simulink model "Week10_Simulation_Trajectory"  (R2017b)
settings: Solver=ode4  StartTime=0.0  StopTime=20  FixedStep=1e-3  RelTol=1e-3  EnableMultiTasking=on
undefined symbols (not defined in the file): DiscIntNeverNeededParam
libraries: simulink x2
settings Model: Creator=e27269  LastModifiedBy=e27269
settings DataIOCC: LimitDataPoints=on
settings OptimizationCC: LifeSpan=inf
settings DebuggingCC: AllowSymbolicDim=off  SFUnexpectedBacktrackingDiag=warning  SFNoUnconditionalDefaultTransitionDiag=warning  SFExecutionAtInitializationDiag=none
settings ModelReferenceCC: PropagateSignalLabelsOutOfModel=off
settings CodeAppCC: StateflowObjectComments=on
settings GRTTargetCC: TargetLangStandard=C89/C90 (ANSI)
settings ConfigComp: CovMetricSettings=dw  CovHtmlReporting=on  CovSaveCumulativeToWorkspaceVar=on  CovSaveSingleToWorkspaceVar=on  CovExternalEMLEnable=off

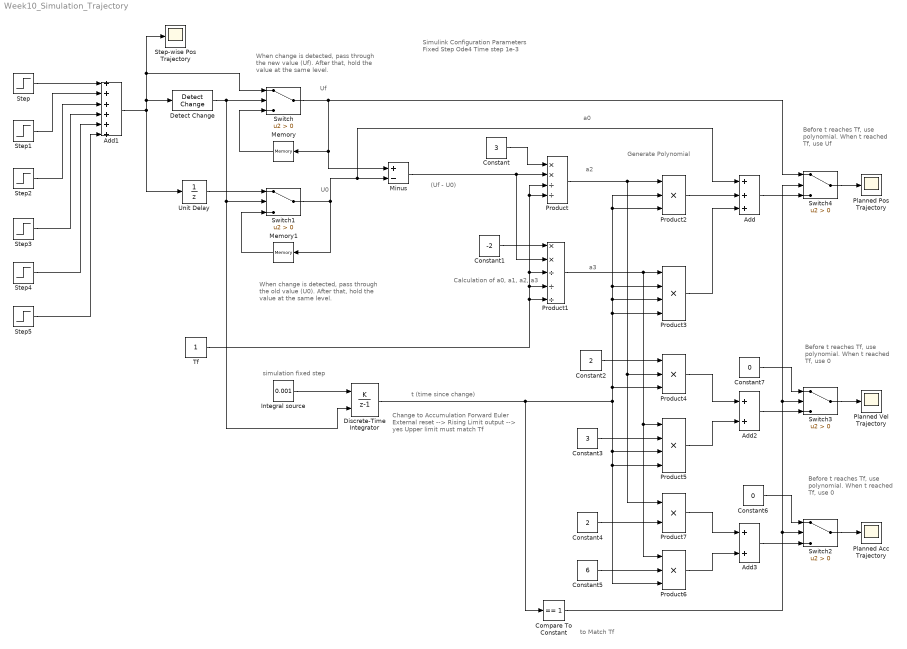
== system Week10_Simulation_Trajectory ==
  note: Generate Polynomial
  note: Calculation of
      | a0, a1, a2, a3
  note: Before t reaches Tf,
      | use polynomial.
      | When t reached Tf,
      | use Uf
  note: to Match Tf
  note: t (time since change)
  note: (Uf - U0)
  note: When change is detected, pass through
      | the old value (U0). After that, hold the
      | value at the same level.
  note: Simulink Configuration Parameters
      | Fixed Step
      | Ode4
      | Time step 1e-3
  note: simulation fixed step
  note: Change to Accumulation Forward Euler
      | External reset --> Rising
      | Limit output --> yes
      | Upper limit must match Tf
  note: a0
  note: a3
  note: a2
  note: Uf
  note: U0
  note: When change is detected, pass through
      | the new value (Uf). After that, hold the
      | value at the same level.
  note: Before t reaches Tf,
      | use polynomial.
      | When t reached Tf,
      | use 0
  note: Before t reaches Tf,
      | use polynomial.
      | When t reached Tf,
      | use 0
  Add : Sum  Inputs=3
  Add1 : Sum  Inputs=6
  Add2 : Sum  Inputs=2
  Add3 : Sum  Inputs=2
  Compare To Constant : simulink/Logic and Bit Operations/Compare To Constant  relop===  const=1  OutDataTypeStr=boolean
  Constant : Constant  Value=3
  Constant1 : Constant  Value=-2
  Constant2 : Constant  Value=2
  Constant3 : Constant  Value=3
  Constant4 : Constant  Value=2
  Constant5 : Constant  Value=6
  Constant6 : Constant  Value=0
  Constant7 : Constant  Value=0
  Detect Change : simulink/Logic and Bit Operations/Detect Change  vinit=0  InputProcessing=Inherited  OutDataTypeStr=boolean
  Discrete-Time Integrator : DiscreteIntegrator  IntegratorMethod=Accumulation: Forward Euler  gainval=1  ExternalReset=rising  InitialConditionSetting=State (most efficient)  SampleTime=-1  LimitOutput=on  UpperSaturationLimit=1  ICPrevOutput=DiscIntNeverNeededParam  ICPrevScaledInput=DiscIntNeverNeededParam
  Integral source : Constant  Value=0.001
  Memory : Memory  InheritSampleTime=on
  Memory1 : Memory  InheritSampleTime=on
  Minus : Sum  Inputs=+-
  Planned Acc Trajectory : Scope
  Planned Pos Trajectory : Scope
  Planned Vel Trajectory : Scope
  Product : Product  Inputs=**//
  Product1 : Product  Inputs=**///
  Product2 : Product  Inputs=3
  Product3 : Product  Inputs=4
  Product4 : Product  Inputs=3
  Product5 : Product  Inputs=4
  Product6 : Product  Inputs=3
  Product7 : Product
  Step : Step  SampleTime=0
  Step-wise Pos Trajectory : Scope
  Step1 : Step  Time=4  After=2  SampleTime=0
  Step2 : Step  Time=8  After=-1  SampleTime=0
  Step3 : Step  Time=11  After=1.5  SampleTime=0
  Step4 : Step  Time=14  After=-1  SampleTime=0
  Step5 : Step  Time=17  After=-2  SampleTime=0
  Switch{,1..4} (5 alike) : Switch  Criteria=u2 > Threshold
  Tf : Constant
  Unit Delay : UnitDelay  SampleTime=-1
  wires:
  Switch/1 -> Minus/1, Memory/1, Switch4/1
  Memory/1 -> Switch/3
  Unit Delay/1 -> Switch1/1
  Switch1/1 -> Memory1/1, Add/1, Minus/2
  Memory1/1 -> Switch1/3
  Minus/1 -> Product1/2, Product/2
  Constant/1 -> Product/1
  Tf/1 -> Product1/5, Product1/4, Product1/3, Product/4, Product/3
  Product/1 -> Product7/1, Product4/2, Product2/1
  Constant1/1 -> Product1/1
  Product1/1 -> Product6/1, Product5/1, Product3/1
  Integral source/1 -> Discrete-Time Integrator/1
  Discrete-Time Integrator/1 -> Compare To Constant/1, Product5/3, Product6/3, Product5/4, Product4/3, Product3/4, Product3/3, Product3/2, Product2/3, Product2/2
  Product2/1 -> Add/2
  Product3/1 -> Add/3
  Detect Change/1 -> Discrete-Time Integrator/2, Switch1/2, Switch/2
  Add1/1 -> Switch/1, Step-wise Pos Trajectory/1, Detect Change/1, Unit Delay/1
  Step/1 -> Add1/1
  Step1/1 -> Add1/2
  Step2/1 -> Add1/3
  Step3/1 -> Add1/4
  Step4/1 -> Add1/5
  Step5/1 -> Add1/6
  Constant2/1 -> Product4/1
  Constant3/1 -> Product5/2
  Product5/1 -> Add2/2
  Product4/1 -> Add2/1
  Constant4/1 -> Product7/2
  Constant5/1 -> Product6/2
  Product6/1 -> Add3/2
  Product7/1 -> Add3/1
  Add3/1 -> Switch2/3
  Switch2/1 -> Planned Acc Trajectory/1
  Constant6/1 -> Switch2/1
  Compare To Constant/1 -> Switch4/2, Switch3/2, Switch2/2
  Add2/1 -> Switch3/3
  Switch3/1 -> Planned Vel Trajectory/1
  Add/1 -> Switch4/3
  Switch4/1 -> Planned Pos Trajectory/1
  Constant7/1 -> Switch3/1
